simulink model "aeromissile_la"  (R2019b)
settings: Solver=ode45  StartTime=0.0  StopTime=20  RelTol=1e-3  EnableMultiTasking=on
PreLoadFcn:
  | aeromissile_la_dat
values from neighbouring files (symbols this model uses):
  cy_el = 0.034000/d2r    (= 1.94805650344)    [aeromissile_la_dat.m]
  cz_el = -0.034000/d2r    (= -1.94805650344)    [aeromissile_la_dat.m]
  d_ref = 0.2286    [aeromissile_la_dat.m]
  eul_0 = [0;0;0]    [aeromissile_la_dat.m]
  fin_max = 30.0*d2r    (= 0.523598775598)    [aeromissile_la_dat.m]
  fin_min = -30.0*d2r    (= -0.523598775598)    [aeromissile_la_dat.m]
  g = 9.81    [aeromissile_la_dat.m]
  inertia = inertia_0/2    [aeromissile_la_dat.m]
  inertia_0 = diag([Ixx Iyy Izz])    [aeromissile_la_dat.m]
  l_acc = 0.5    [aeromissile_la_dat.m]
  l_ref = 0.04    [aeromissile_la_dat.m]
  len_missile = 3    [aeromissile_la_dat.m]
  mass_0 = 234.02    [aeromissile_la_dat.m]
  massf = 30    [aeromissile_la_dat.m]
  mx_el = -0.206000/d2r    (= -11.8029305797)    [aeromissile_la_dat.m]
  mx_wx = -0.5    [aeromissile_la_dat.m]
  my_el = -0.206000/d2r    (= -11.8029305797)    [aeromissile_la_dat.m]
  my_wy = -1.719    [aeromissile_la_dat.m]
  mz_el = -0.206000/d2r    (= -11.8029305797)    [aeromissile_la_dat.m]
  mz_wz = -1.719    [aeromissile_la_dat.m]
  q = 2    [aeromissile_la_dat.m]
  S_ref = 0.040877    [aeromissile_la_dat.m]
  Thrust = 10e3    (= 10000)    [aeromissile_la_dat.m]
  Vm_0 = [300;0;0]    [aeromissile_la_dat.m]
  wm_0 = [0;0;0]    [aeromissile_la_dat.m]
  x_cg = 0.555*len_missile    (= 1.665)    [aeromissile_la_dat.m]
  x_cg_0 = 0.575*len_missile    (= 1.725)    [aeromissile_la_dat.m]
  x_ref = 0.54*len_missile    (= 1.62)    [aeromissile_la_dat.m]
  xmg_0 = [0;1000;0]    [aeromissile_la_dat.m]
undefined symbols (not defined in the file or in its folder): Earth, inv_fcn, WGS84
libraries: simulink_need_slupdate x26, sharedutil x3, aerolibobsolete x2, aerolibtransform2 x2, aerolibfltsims x2, aerolibprivatev1p5 x1, vrlib x1
(part 1 of 2)
settings Model: EnablePacing=on  Creator=Semen  LastModifiedBy=Semen
settings DataIOCC: LimitDataPoints=on  SaveFormat=Array  ReturnWorkspaceOutputs=off  SignalLoggingName=sigsOut
settings DebuggingCC: SaveWithParameterizedLinksMsg=none  UnderspecifiedInitializationDetection=Classic  MergeDetectMultiDrivingBlocksExec=none  SignalResolutionControl=TryResolveAllWithWarning  MultiTaskDSMMsg=warning  MultiTaskCondExecSysMsg=none
settings HardwareCC: ProdBitPerPointer=32  ProdBitPerSizeT=32  ProdBitPerPtrDiffT=32  ProdLargestAtomicFloat=None  ProdIntDivRoundTo=Undefined  ProdEndianess=Unspecified  ProdWordSize=32  ProdHWDeviceType=32-bit Generic  TargetUnknown=on
settings ModelReferenceCC: PropagateSignalLabelsOutOfModel=off
settings GRTTargetCC: CombineOutputUpdateFcns=off  GRTInterface=on
settings ConfigComp: CovMetricSettings=dw  CovHtmlReporting=on  CovSaveCumulativeToWorkspaceVar=on  CovSaveSingleToWorkspaceVar=on

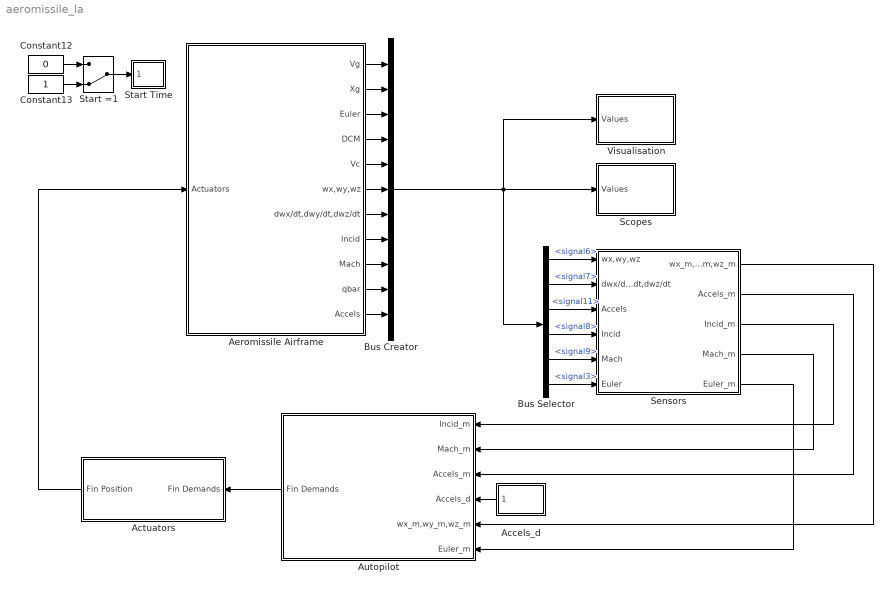
== system aeromissile_la ==
  Accels_d : Subsystem
  Actuators : Subsystem
  Aeromissile Airframe : Subsystem
  Autopilot : Subsystem
  Bus Creator : BusCreator  Inputs=11
  Bus Selector : BusSelector  OutputSignals=signal6,signal7,signal11,signal8,signal9,signal3
  Constant12 : Constant  Value=0  VectorParams1D=off
  Constant13 : Constant  VectorParams1D=off
  Scopes : Subsystem
  Sensors : Subsystem
  Start =1 : ManualSwitch  CurrentSetting=0
  Start Time : Subsystem
  Visualisation : Subsystem
  wires:
  Sensors/1(wx_m,wy_m,wz_m) -> Autopilot/5(wx_m,wy_m,wz_m)
  Sensors/2(Accels_m) -> Autopilot/3(Accels_m)
  Aeromissile Airframe/1(Vg) -> Bus Creator/1
  Aeromissile Airframe/2(Xg) -> Bus Creator/2
  Aeromissile Airframe/3(Euler) -> Bus Creator/3
  Aeromissile Airframe/4(DCM) -> Bus Creator/4
  Aeromissile Airframe/5(Vc) -> Bus Creator/5
  Aeromissile Airframe/6(wx,wy,wz) -> Bus Creator/6
  Aeromissile Airframe/7(dwx/dt,dwy/dt,dwz/dt) -> Bus Creator/7
  Aeromissile Airframe/11(Accels) -> Bus Creator/11
  Bus Selector/1 -> Sensors/1(wx,wy,wz)  "<signal6>"
  Bus Selector/2 -> Sensors/2(dwx/dt,dwy/dt,dwz/dt)  "<signal7>"
  Bus Selector/3 -> Sensors/3(Accels)  "<signal11>"
  Aeromissile Airframe/8(Incid) -> Bus Creator/8
  Aeromissile Airframe/10(qbar) -> Bus Creator/10
  Actuators/1(Fin Position) -> Aeromissile Airframe/1(Actuators)
  Sensors/3(Incid_m) -> Autopilot/1(Incid_m)
  Sensors/4(Mach_m) -> Autopilot/2(Mach_m)
  Bus Selector/4 -> Sensors/4(Incid)  "<signal8>"
  Bus Selector/5 -> Sensors/5(Mach)  "<signal9>"
  Bus Selector/6 -> Sensors/6(Euler)  "<signal3>"
  Sensors/5(Euler_m) -> Autopilot/6(Euler_m)
  Constant13/1 -> Start =1/2
  Constant12/1 -> Start =1/1
  Bus Creator/1 -> Visualisation/1(Values), Scopes/1(Values), Bus Selector/1
  Aeromissile Airframe/9(Mach) -> Bus Creator/9
  Start =1/1 -> Start Time/1(Start)
  Autopilot/1(Fin Demands) -> Actuators/1(Fin Demands)
  Accels_d/1("Accels_d ") -> Autopilot/4(Accels_d)

== system aeromissile_la/Accels_d ==
  Accels_d : Constant  Value=[0 g 1]  VectorParams1D=off
  Accels_dD : Constant  Value=[0 0 0]  VectorParams1D=off
  Switch : Switch  Criteria=u2 ~= 0  SaturateOnIntegerOverflow=on
  "Accels_d " : Outport
  wires:
  Switch/1 -> "Accels_d "/1
  Accels_dD/1 -> Switch/3
  [tD] -> Switch/2
  Accels_d/1 -> Switch/1

== system aeromissile_la/Actuators ==
  Fin Demands : Inport
  Lock Fin : Subsystem
  Second Order Nonlinear Actuator : aerolibobsolete/Second Order Nonlinear Actuator  wn_fin=wn_fin  z_fin=z_fin  fin_max=fin_max  fin_min=fin_min  fin_maxrate=fin_maxrate  fin_act_0=fin_act_0
      settings: SourceProductName=Aerospace Blockset  SourceProductBaseCode=AE
  Fin Position : Outport
  wires:
  Fin Demands/1 -> Lock Fin/1(FD)
  Second Order Nonlinear Actuator/1 -> Fin Position/1
  Lock Fin/1("FD ") -> Second Order Nonlinear Actuator/1

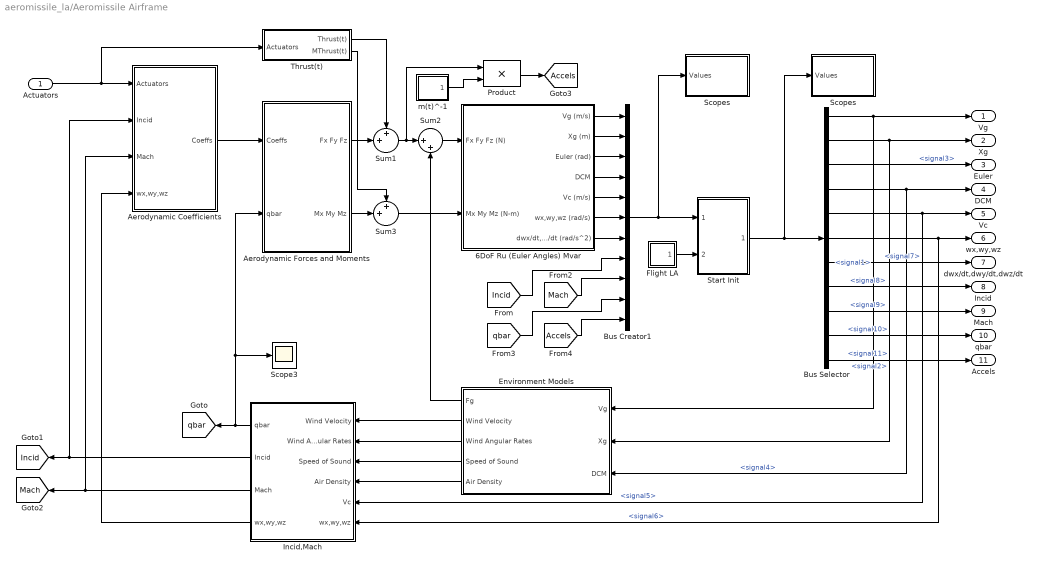
== system aeromissile_la/Aeromissile Airframe ==
  Actuators : Inport
  6DoF Ru (Euler Angles) Mvar : Subsystem  AncestorBlock=aerolib6dof/6DoF (Euler Angles)  mask(6DoF Ru (Euler Angles) EoM){xmg_0=xmg_0, Vm_0=Vm_0, eul_0=eul_0, wm_0=wm_0, mass_0=mass_0, massf=massf, q=q, inertia_0=inertia_0, inertia=inertia}
      mask prompts: xmg_0 "Initial position in inertial axes [Xg,Yg,Zg] (m):"; Vm_0 "Initial velocity in body axes [Vxc,Vyc,Vzc] (m/s):"; eul_0 "Initial Euler orientation [roll, pitch, yaw] (rad):"; wm_0 "Initial body rotation rates [wx,wy,wz] (rad/s):"; mass_0 "Initial mass(kg):"; massf "Mass of fuel (kg):"; q "Consumption of fuel (kg/s):"; inertia_0 "Initial inertia matrix (kg*m^2):"; inertia "Finite inertia matrix (kg*m^2)"
      mask help:
      | Integrate the six-degrees-of-freedom equations of motion using an Euler angle representation for the orientation of the body in space.
      |
      | Inputs are forces on the body in x-axis, y-axis, and z-axis; and moments on the body along x-axis, y-axis, and z-axis. Outputs are translational velocity in x-axis, y-axis, and z-axis in inertial coordinates; position in x-axis, y-axis, and z-axis in inertial coordinates; gamma, theta, and psi; 3-by-3 direction cosine matrix; translational velocity in x-axis, y-axis, and z-axis in body coordinates; roll, pitch, and yaw rate; and roll, pitch, and yaw acceleration.
      mask Display: disp('Euler\nAngles')
  Aerodynamic Coefficients : Subsystem
  Aerodynamic Forces and Moments : Subsystem  AncestorBlock=aeroblk_lib_HL20/HL20 Airframe/Forces and Moments
  Bus Creator1 : BusCreator  Inputs=11
  Bus Selector : BusSelector  OutputSignals=signal1,signal2,signal3,signal4,signal5,signal6,signal7,signal8,signal9,signal10,signal11
  Environment Models : Subsystem
  Flight LA : Subsystem
  Incid,Mach : Subsystem
  Product : Product  SaturateOnIntegerOverflow=on  OutDataTypeStr=Inherit: Same as first input
  Scope3 : Scope
  Scopes : Subsystem
  "Scopes " : Subsystem
  Start Init : Subsystem
  Sum1 : Sum  Inputs=++|  SaturateOnIntegerOverflow=on
  Sum2 : Sum  Inputs=|++  SaturateOnIntegerOverflow=on
  Sum3 : Sum  Inputs=++|  SaturateOnIntegerOverflow=on
  Thrust(t) : Subsystem
  m(t)^-1 : Subsystem
  Vg : Outport
  Xg : Outport  Port=2
  Euler : Outport  Port=3
  DCM : Outport  Port=4
  Vc : Outport  Port=5
  wx,wy,wz : Outport  Port=6
  dwx/dt,dwy/dt,dwz/dt : Outport  Port=7
  Incid : Outport  Port=8
  Mach : Outport  Port=9
  qbar : Outport  Port=10
  Accels : Outport  Port=11
  tag scope: Accels=global, Incid=global, Mach=global, qbar=global
  wires:
  Aerodynamic Coefficients/1(Coeffs) -> Aerodynamic Forces and Moments/1(Coeffs)
  Actuators/1 -> Aerodynamic Coefficients/1(Actuators), Thrust(t)/1(Actuators)
  Environment Models/1(Fg) -> Sum2/2
  Incid,Mach/1(qbar) -> Aerodynamic Forces and Moments/2(qbar), Scope3/1, [qbar]
  Incid,Mach/2(Incid) -> Aerodynamic Coefficients/2(Incid), [Incid]
  Incid,Mach/3(Mach) -> Aerodynamic Coefficients/3(Mach), [Mach]
  Incid,Mach/4("wx,wy,wz ") -> Aerodynamic Coefficients/4(wx,wy,wz)
  Environment Models/2(Wind Velocity) -> Incid,Mach/1(Wind Velocity)
  Environment Models/3(Wind Angular Rates) -> Incid,Mach/2(Wind Angular Rates)
  Environment Models/4(Speed of Sound) -> Incid,Mach/3(Speed of Sound)
  Environment Models/5(Air Density) -> Incid,Mach/4(Air Density)
  Aerodynamic Forces and Moments/1(Fx Fy Fz) -> Sum1/2
  Sum1/1 -> Sum2/1, Product/1
  m(t)^-1/1(m(t)^-1) -> Product/2
  6DoF Ru (Euler Angles) Mvar/1(Vg (m/s)) -> Bus Creator1/1
  6DoF Ru (Euler Angles) Mvar/2(Xg (m)) -> Bus Creator1/2
  6DoF Ru (Euler Angles) Mvar/3(Euler (rad)) -> Bus Creator1/3
  6DoF Ru (Euler Angles) Mvar/4(DCM) -> Bus Creator1/4
  6DoF Ru (Euler Angles) Mvar/5(Vc (m/s)) -> Bus Creator1/5
  6DoF Ru (Euler Angles) Mvar/6(wx,wy,wz (rad/s)) -> Bus Creator1/6
  6DoF Ru (Euler Angles) Mvar/7(dwx/dt,dwy/dt,dwz/dt (rad/s^2)) -> Bus Creator1/7
  Bus Selector/1 -> Vg/1, Environment Models/1(Vg)  "<signal1>"
  Bus Selector/2 -> Xg/1, Environment Models/2(Xg)  "<signal2>"
  Bus Selector/3 -> Euler/1  "<signal3>"
  Bus Selector/4 -> DCM/1, Environment Models/3(DCM)  "<signal4>"
  Bus Selector/5 -> Vc/1, Incid,Mach/5(Vc)  "<signal5>"
  Bus Selector/6 -> wx,wy,wz/1, Incid,Mach/6(wx,wy,wz)  "<signal6>"
  Bus Selector/7 -> dwx/dt,dwy/dt,dwz/dt/1  "<signal7>"
  Product/1 -> [Accels]
  Bus Selector/8 -> Incid/1  "<signal8>"
  Bus Selector/9 -> Mach/1  "<signal9>"
  Bus Selector/10 -> qbar/1  "<signal10>"
  Bus Selector/11 -> Accels/1  "<signal11>"
  [Incid] -> Bus Creator1/8
  [Mach] -> Bus Creator1/9
  [qbar] -> Bus Creator1/10
  [Accels] -> Bus Creator1/11
  Bus Creator1/1 -> Start Init/1("val_m "), Scopes/1(Values)
  Start Init/1(val_m) -> Bus Selector/1, "Scopes "/1(Values)
  Flight LA/1(val_la) -> Start Init/2("val_la ")
  Sum2/1 -> 6DoF Ru (Euler Angles) Mvar/1(Fx Fy Fz (N))
  Aerodynamic Forces and Moments/2(Mx My Mz) -> Sum3/2
  Sum3/1 -> 6DoF Ru (Euler Angles) Mvar/2(Mx My Mz (N-m))
  Thrust(t)/2(MThrust(t)) -> Sum3/1
  Thrust(t)/1(Thrust(t)) -> Sum1/1

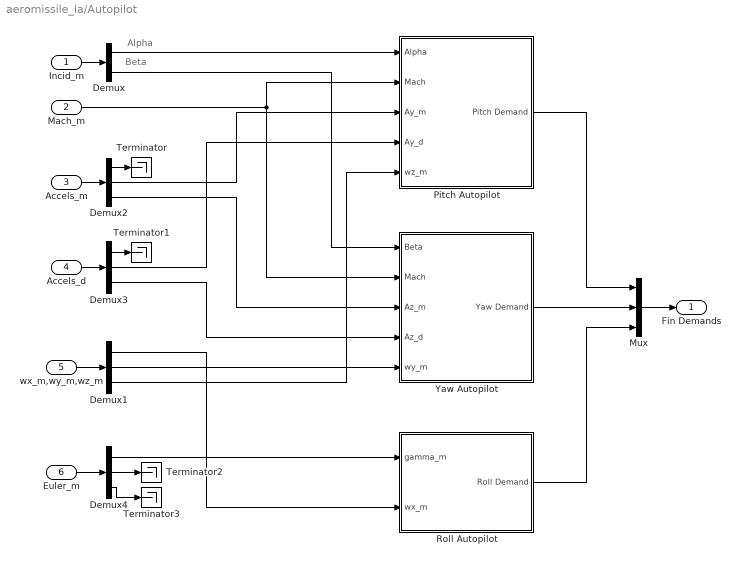
== system aeromissile_la/Autopilot ==
  note: Alpha
  note: Beta
  Incid_m : Inport
  Mach_m : Inport  Port=2
  Accels_m : Inport  Port=3
  Accels_d : Inport  Port=4
  wx_m,wy_m,wz_m : Inport  Port=5
  Euler_m : Inport  Port=6
  Demux : Demux  Outputs=2
  Demux{1..4} (4 alike) : Demux  Outputs=3
  Mux : Mux  Inputs=3
  Pitch Autopilot : Subsystem
  Roll Autopilot : Subsystem
  Terminator{,1..3} (4 alike) : Terminator
  Yaw Autopilot : Subsystem
  Fin Demands : Outport
  wires:
  Accels_m/1 -> Demux2/1
  Accels_d/1 -> Demux3/1
  Demux2/1 -> Terminator/1
  Demux3/1 -> Terminator1/1
  Incid_m/1 -> Demux/1
  Demux/1 -> Pitch Autopilot/1(Alpha)
  Demux/2 -> Yaw Autopilot/1(Beta)
  Demux2/2 -> Pitch Autopilot/3(Ay_m)
  Demux2/3 -> Yaw Autopilot/3(Az_m)
  Demux3/2 -> Pitch Autopilot/4(Ay_d)
  wx_m,wy_m,wz_m/1 -> Demux1/1
  Demux1/3 -> Pitch Autopilot/5(wz_m)
  Mach_m/1 -> Pitch Autopilot/2(Mach), Yaw Autopilot/2(Mach)
  Demux1/1 -> Roll Autopilot/2(wx_m)
  Demux3/3 -> Yaw Autopilot/4(Az_d)
  Demux1/2 -> Yaw Autopilot/5(wy_m)
  Pitch Autopilot/1(Pitch Demand) -> Mux/1
  Yaw Autopilot/1(Yaw Demand) -> Mux/2
  Roll Autopilot/1(Roll Demand) -> Mux/3
  Mux/1 -> Fin Demands/1
  Euler_m/1 -> Demux4/1
  Demux4/2 -> Terminator2/1
  Demux4/3 -> Terminator3/1
  Demux4/1 -> Roll Autopilot/1(gamma_m)

== system aeromissile_la/Scopes ==
  note: Vg
  note: Xg
  note: Euler
  note: DCM
  note: Vc
  note: wx,wy,wz
  note: dwx/dt,dwy/dt,
      | dwz/dt
  note: Incid
  note: Mach
  note: qbar
  note: Accels
  Values : Inport
  Bus Selector : BusSelector  OutputSignals=signal1,signal2,signal3,signal4,signal5,signal6,signal7,signal8,signal9,signal10,signal11
  Scope{1..11} (11 alike) : Scope
  wires:
  Bus Selector/1 -> Scope2/1  "<signal1>"
  Bus Selector/2 -> Scope1/1  "<signal2>"
  Bus Selector/3 -> Scope4/1  "<signal3>"
  Bus Selector/11 -> Scope11/1  "<signal11>"
  Bus Selector/10 -> Scope10/1  "<signal10>"
  Bus Selector/9 -> Scope9/1  "<signal9>"
  Bus Selector/8 -> Scope8/1  "<signal8>"
  Bus Selector/7 -> Scope7/1  "<signal7>"
  Bus Selector/6 -> Scope6/1  "<signal6>"
  Bus Selector/5 -> Scope5/1  "<signal5>"
  Bus Selector/4 -> Scope3/1  "<signal4>"
  Values/1 -> Bus Selector/1

== system aeromissile_la/Sensors ==
  note: Rate Gyro
  wx,wy,wz : Inport
  dwx/dt,dwy/dt,dwz/dt : Inport  Port=2
  Accels : Inport  Port=3
  Incid : Inport  Port=4
  Mach : Inport  Port=5
  Euler : Inport  Port=6
  Demux : Demux  Outputs=3
  Demux1 : Demux  Outputs=3
  Gain : Gain  Gain=l_acc  SaturateOnIntegerOverflow=on  OutDataTypeStr=Inherit: Same as input  ParamDataTypeStr=Inherit: Same as input
  Mux : Mux  Inputs=3
  Sum : Sum  Inputs=-+|  SaturateOnIntegerOverflow=on
  Sum1 : Sum  Inputs=++|  SaturateOnIntegerOverflow=on
  Tminator1 : Terminator
  wx_m,wy_m,wz_m : Outport
  Accels_m : Outport  Port=2
  Incid_m : Outport  Port=3
  Mach_m : Outport  Port=4
  Euler_m : Outport  Port=5
  wires:
  wx,wy,wz/1 -> wx_m,wy_m,wz_m/1
  dwx/dt,dwy/dt,dwz/dt/1 -> Gain/1
  Accels/1 -> Demux/1
  Demux/1 -> Mux/1
  Gain/1 -> Demux1/1
  Demux/3 -> Sum/2
  Demux1/2 -> Sum/1
  Demux1/1 -> Tminator1/1
  Sum/1 -> Mux/3
  Mux/1 -> Accels_m/1  "Accelerometer"
  Demux/2 -> Sum1/2
  Demux1/3 -> Sum1/1
  Sum1/1 -> Mux/2
  Incid/1 -> Incid_m/1
  Mach/1 -> Mach_m/1
  Euler/1 -> Euler_m/1

== system aeromissile_la/Start Time ==
  Start : Inport
  t departure : Subsystem
  t engine : Subsystem
  t start : Subsystem
  tag scope: Start=global, tD=global, tE=global, tS=global
  wires:
  t start/1(tS) -> t engine/1(tS), [tS], t departure/1(tS)
  t engine/1(tE) -> [tE]
  t departure/1(tD) -> [tD]
  Start/1 -> t start/1(S), [Start]

== system aeromissile_la/Visualisation ==
  note: Euler
  note: Xg
  Values : Inport
  Bus Selector : BusSelector  OutputSignals=signal2,signal3
  FlightGear Animation : Subsystem
  Scope1 : Scope
  Scope4 : Scope
  VR Sink Animation : Subsystem
  wires:
  Bus Selector/2 -> FlightGear Animation/2(Euler), Scope4/1, VR Sink Animation/2(Euler)  "<signal3>"
  Bus Selector/1 -> VR Sink Animation/1(Xg), FlightGear Animation/1(Xg), Scope1/1  "<signal2>"
  Values/1 -> Bus Selector/1

== system aeromissile_la/Actuators/Lock Fin ==
  FD : Inport
  Constant6 : Constant  Value=[0; 0; 0]  VectorParams1D=off
  Switch : Switch  Criteria=u2 ~= 0  SaturateOnIntegerOverflow=on
  "FD " : Outport
  wires:
  FD/1 -> Switch/1
  Switch/1 -> "FD "/1
  [Start] -> Switch/2
  Constant6/1 -> Switch/3

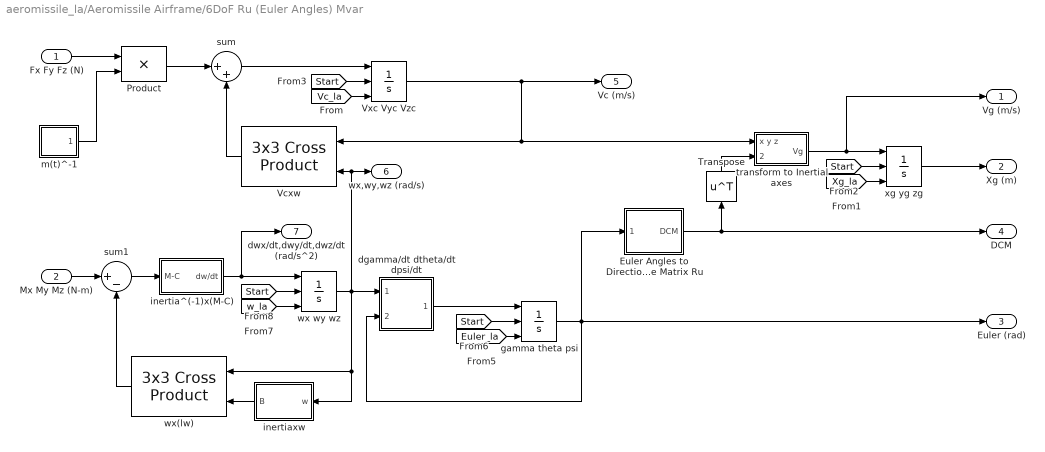
== system aeromissile_la/Aeromissile Airframe/6DoF Ru (Euler Angles) Mvar ==
  Fx Fy Fz (N) : Inport
  Mx My Mz (N-m) : Inport  Port=2
  Euler Angles to Direction Cosine Matrix Ru : Subsystem  AncestorBlock="aerolibtransform/Euler Angles to  Direction Cosine Matrix"  mask(Euler2DCM){}
      mask help: Determine the 3-by-3 direction cosine matrix (DCM) from an Euler orientation (roll, pitch, yaw). The output DCM transforms vectors from inertial axes to body axes.
      mask Help: web(asbhelp('euleranglestodirectioncosinematrix'));
      mask Display: disp('Eul2DCM')
  Product : Product  SaturateOnIntegerOverflow=on  OutDataTypeStr=Inherit: Same as first input
  Transpose : Math  Operator=transpose  SaturateOnIntegerOverflow=on
  Vcxw : sharedutil/3x3 Cross Product  aMode=aMode
      settings: SourceProductBaseCode=AE
  Vxc Vyc Vzc : Integrator  ExternalReset=either  InitialConditionSource=external  InitialCondition=Vm_0
  dgamma/dt dtheta/dt dpsi/dt : Subsystem
  gamma theta psi : Integrator  ExternalReset=either  InitialConditionSource=external  InitialCondition=Vm_0
  inertia^(-1)x(M-C) : Subsystem
  inertiaxw : Subsystem
  m(t)^-1 : Subsystem
  sum : Sum  Inputs=|++  SaturateOnIntegerOverflow=on  InputSameDT=on  OutDataTypeStr=Inherit: Same as first input
  sum1 : Sum  Inputs=|+-  SaturateOnIntegerOverflow=on  InputSameDT=on  OutDataTypeStr=Inherit: Same as first input
  "transform to Inertial axes " : Subsystem  mask(Vector Transformation){}
      mask Display: disp('L_EB')
  wx wy wz : Integrator  ExternalReset=either  InitialConditionSource=external  InitialCondition=Vm_0
  wx(lw) : sharedutil/3x3 Cross Product  aMode=aMode
      settings: SourceProductBaseCode=AE
  xg yg zg : Integrator  ExternalReset=either  InitialConditionSource=external  InitialCondition=Vm_0
  Vg (m/s) : Outport
  Xg (m) : Outport  Port=2
  Euler (rad) : Outport  Port=3
  DCM : Outport  Port=4
  Vc (m/s) : Outport  Port=5
  wx,wy,wz (rad/s) : Outport  Port=6
  dwx/dt,dwy/dt,dwz/dt (rad/s^2) : Outport  Port=7
  wires:
  Transpose/1 -> "transform to Inertial axes "/2(transform coefficients)
  Euler Angles to Direction Cosine Matrix Ru/1(DCM) -> Transpose/1, DCM/1
  Product/1 -> sum/1
  Vcxw/1 -> sum/2
  Fx Fy Fz (N)/1 -> Product/1
  inertia^(-1)x(M-C)/1(dw/dt) -> dwx/dt,dwy/dt,dwz/dt (rad/s^2)/1, wx wy wz/1
  wx(lw)/1 -> sum1/2
  inertiaxw/1(B) -> wx(lw)/2
  Mx My Mz (N-m)/1 -> sum1/1
  sum1/1 -> inertia^(-1)x(M-C)/1(M-C)
  wx wy wz/1 -> Vcxw/2, wx,wy,wz (rad/s)/1, wx(lw)/1, inertiaxw/1(w), dgamma/dt dtheta/dt dpsi/dt/1(wx wy wz)
  "transform to Inertial axes "/1(Vg) -> Vg (m/s)/1, xg yg zg/1
  xg yg zg/1 -> Xg (m)/1
  Vxc Vyc Vzc/1 -> "transform to Inertial axes "/1(x y z), Vcxw/1, Vc (m/s)/1
  gamma theta psi/1 -> dgamma/dt dtheta/dt dpsi/dt/2(gamma theta psi), Euler Angles to Direction Cosine Matrix Ru/1(Euler Roll Pitch Yaw), Euler (rad)/1
  dgamma/dt dtheta/dt dpsi/dt/1(dgamma/dt dtheta/dt dpsi/dt) -> gamma theta psi/1
  m(t)^-1/1(m(t)^-1) -> Product/2
  [Start] -> xg yg zg/2
  [Xg_la] -> xg yg zg/3
  sum/1 -> Vxc Vyc Vzc/1
  [Start] -> Vxc Vyc Vzc/2
  [Vc_la] -> Vxc Vyc Vzc/3
  [Euler_la] -> gamma theta psi/3
  [Start] -> wx wy wz/2
  [w_la] -> wx wy wz/3
  [Start] -> gamma theta psi/2

== system aeromissile_la/Aeromissile Airframe/Aerodynamic Coefficients ==
  Actuators : Inport
  Incid : Inport  Port=2
  Mach : Inport  Port=3
  wx,wy,wz : Inport  Port=4
  Actuator Increments : Subsystem
  Body Rate Damping : Subsystem
  Cross Link Coefficients : Subsystem
  Datum Coefficients : Subsystem
  Sum : Sum  Inputs=++++  SaturateOnIntegerOverflow=on
  Coeffs : Outport  InitialOutput=[0]
  wires:
  Mach/1 -> Datum Coefficients/2(Mach), Cross Link Coefficients/2(Mach)
  Actuators/1 -> Actuator Increments/1(Actuator Deflections), Cross Link Coefficients/3(Actuators)
  Incid/1 -> Datum Coefficients/1(Incid), Cross Link Coefficients/1(Incid)
  Datum Coefficients/1(Datum Coeffs) -> Sum/1
  Actuator Increments/1(Actuator Coeffs) -> Sum/2
  Sum/1 -> Coeffs/1
  wx,wy,wz/1 -> Body Rate Damping/1(wx,wy,wz)
  Body Rate Damping/1(Damping Coeffs) -> Sum/4
  Cross Link Coefficients/1(Cross Coeffs) -> Sum/3

== system aeromissile_la/Aeromissile Airframe/Aerodynamic Forces and Moments ==
  Coeffs : Inport
  qbar : Inport  Port=2
  3x3 Cross Product : sharedutil/3x3 Cross Product  aMode=aMode
      settings: SourceProductBaseCode=AE
  Demux1 : Demux  Outputs=[3,3]
  Gain : Gain  Gain=[-1 1 1]  SaturateOnIntegerOverflow=on  OutDataTypeStr=Inherit: Same as input  ParamDataTypeStr=Inherit: Same as input
  Moments about Centre of Gravity : Subsystem
  Product : Product  SaturateOnIntegerOverflow=on  InputSameDT=on  OutDataTypeStr=Inherit: Same as first input
  Product3 : Product  SaturateOnIntegerOverflow=on  InputSameDT=on  OutDataTypeStr=Inherit: Same as first input
  Scope : Scope
  Sum1 : Sum  Inputs=++|  SaturateOnIntegerOverflow=on  InputSameDT=on  OutDataTypeStr=Inherit: Same as first input
  reference area : Gain  Gain=S_ref  SaturateOnIntegerOverflow=on  OutDataTypeStr=Inherit: Same as input  ParamDataTypeStr=Inherit: Same as input
  reference length : Gain  Gain=[l_ref d_ref d_ref]  SaturateOnIntegerOverflow=on  OutDataTypeStr=Inherit: Same as input  ParamDataTypeStr=Inherit: Same as input
  Fx Fy Fz : Outport  InitialOutput=[0]
  Mx My Mz : Outport  Port=2  InitialOutput=[0]
  wires:
  Sum1/1 -> Mx My Mz/1
  Product3/1 -> Sum1/2
  Moments about Centre of Gravity/1(-(x_cg-x_ref)) -> 3x3 Cross Product/2, Scope/1
  Product/1 -> 3x3 Cross Product/1, Fx Fy Fz/1
  reference area/1 -> reference length/1, Gain/1
  qbar/1 -> reference area/1
  Demux1/2 -> Product3/1  "mx my mz"
  Demux1/1 -> Product/1  "cx cy cz"
  Coeffs/1 -> Demux1/1
  reference length/1 -> Product3/2
  3x3 Cross Product/1 -> Sum1/1
  Gain/1 -> Product/2

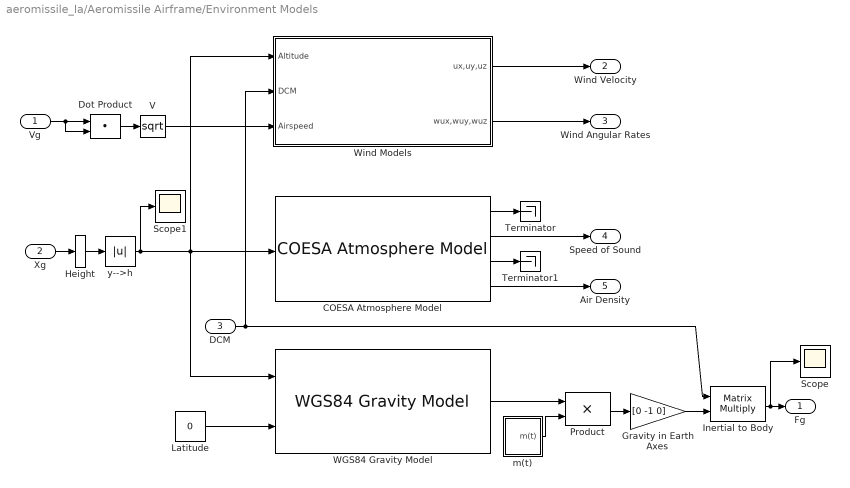
== system aeromissile_la/Aeromissile Airframe/Environment Models ==
  Vg : Inport
  Xg : Inport  Port=2
  DCM : Inport  Port=3
  COESA Atmosphere Model : aerolibprivatev1p5/COESA Atmosphere Model  units=Metric
      settings: SourceProductName=Aerospace Blockset  SourceProductBaseCode=AE
  Dot Product : DotProduct  InputSameDT=on  OutDataTypeStr=Inherit: Inherit via internal rule
  Gravity in Earth Axes : Gain  Gain=[0 -1 0]  SaturateOnIntegerOverflow=on  OutDataTypeStr=Inherit: Same as input  ParamDataTypeStr=Inherit: Same as input
  Height : Selector  InputPortWidth=3  IndexOptions=Index vector (dialog)  Indices=[2]  OutputSizes=1
  Inertial to Body : Product  Multiplication=Matrix(*)  SaturateOnIntegerOverflow=on  InputSameDT=on  OutDataTypeStr=Inherit: Same as first input
  Latitude : Constant  Value=0
  Product : Product  SaturateOnIntegerOverflow=on  OutDataTypeStr=Inherit: Same as first input
  Scope : Scope
  Scope1 : Scope
  Terminator : Terminator
  Terminator1 : Terminator
  V : Math  Operator=sqrt  SaturateOnIntegerOverflow=on
  WGS84 Gravity Model : aerolibobsolete/WGS84 Gravity Model  model=WGS84 Taylor Series  units=Metric (MKS)  no_atmos=on  precessing=on  month=February  day=1  year=2000  no_centrifugal=on  action=Warning
      settings: SourceProductName=Aerospace Blockset  SourceProductBaseCode=AE
  Wind Models : Subsystem
  m(t) : Subsystem
  y-->h : Abs  SaturateOnIntegerOverflow=on
  Fg : Outport
  Wind Velocity : Outport  Port=2
  Wind Angular Rates : Outport  Port=3
  Speed of Sound : Outport  Port=4
  Air Density : Outport  Port=5
  wires:
  Latitude/1 -> WGS84 Gravity Model/2
  COESA Atmosphere Model/1 -> Terminator/1
  COESA Atmosphere Model/3 -> Terminator1/1
  Wind Models/1(ux,uy,uz) -> Wind Velocity/1
  Wind Models/2(wux,wuy,wuz) -> Wind Angular Rates/1
  COESA Atmosphere Model/2 -> Speed of Sound/1
  COESA Atmosphere Model/4 -> Air Density/1
  Height/1 -> y-->h/1
  Xg/1 -> Height/1
  Vg/1 -> Dot Product/2, Dot Product/1
  Dot Product/1 -> V/1
  Gravity in Earth Axes/1 -> Inertial to Body/2
  Inertial to Body/1 -> Fg/1, Scope/1
  DCM/1 -> Wind Models/2(DCM), Inertial to Body/1
  y-->h/1 -> COESA Atmosphere Model/1, WGS84 Gravity Model/1, Wind Models/1(Altitude), Scope1/1
  V/1 -> Wind Models/3(Airspeed)
  WGS84 Gravity Model/1 -> Product/1
  Product/1 -> Gravity in Earth Axes/1
  m(t)/1(m(t)) -> Product/2

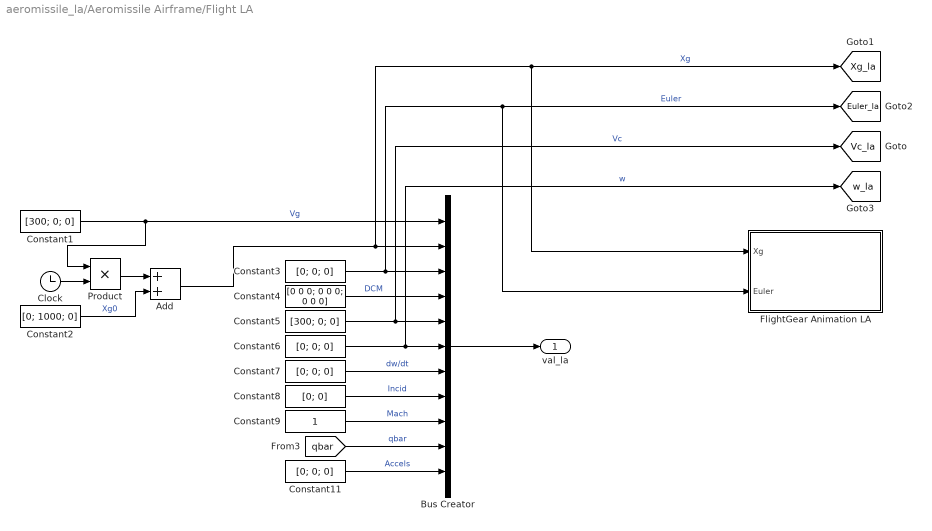
== system aeromissile_la/Aeromissile Airframe/Flight LA ==
  Add : Sum
  Bus Creator : BusCreator  Inputs=11
  Clock : Clock
  Constant1 : Constant  Value=[300; 0; 0]  VectorParams1D=off
  Constant{3,6..7,11} (4 alike) : Constant  Value=[0; 0; 0]  VectorParams1D=off
  Constant2 : Constant  Value=[0; 1000; 0]  VectorParams1D=off
  Constant4 : Constant  Value=[0 0 0; 0 0 0; 0 0 0]  VectorParams1D=off
  Constant5 : Constant  Value=[300; 0; 0]  VectorParams1D=off
  Constant8 : Constant  Value=[0; 0]  VectorParams1D=off
  Constant9 : Constant  VectorParams1D=off
  FlightGear Animation LA : Subsystem
  Product : Product
  val_la : Outport
  tag scope: Euler_la=global, Vc_la=global, Xg_la=global, w_la=global
  wires:
  Constant1/1 -> Product/1, Bus Creator/1  "Vg"
  Constant3/1 -> Bus Creator/3, FlightGear Animation LA/2(Euler), [Euler_la]  "Euler"
  Constant6/1 -> Bus Creator/6, [w_la]  "w"
  Constant7/1 -> Bus Creator/7  "dw/dt"
  Constant8/1 -> Bus Creator/8  "Incid"
  Constant9/1 -> Bus Creator/9  "Mach"
  [qbar] -> Bus Creator/10  "qbar"
  Constant11/1 -> Bus Creator/11  "Accels"
  Bus Creator/1 -> val_la/1
  Constant4/1 -> Bus Creator/4  "DCM"
  Constant5/1 -> Bus Creator/5, [Vc_la]  "Vc"
  Clock/1 -> Product/2
  Constant2/1 -> Add/2  "Xg0"
  Product/1 -> Add/1
  Add/1 -> FlightGear Animation LA/1(Xg), [Xg_la], Bus Creator/2  "Xg"

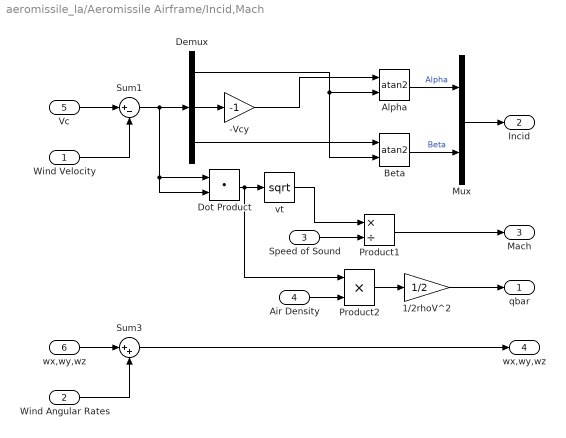
== system aeromissile_la/Aeromissile Airframe/Incid,Mach ==
  Wind Velocity : Inport
  Wind Angular Rates : Inport  Port=2
  Speed of Sound : Inport  Port=3
  Air Density : Inport  Port=4
  Vc : Inport  Port=5
  wx,wy,wz : Inport  Port=6
  -Vcy : Gain  Gain=-1  SaturateOnIntegerOverflow=on  OutDataTypeStr=Inherit: Same as input  ParamDataTypeStr=Inherit: Same as input
  1/2rhoV^2 : Gain  Gain=1/2  SaturateOnIntegerOverflow=on  OutDataTypeStr=Inherit: Same as input  ParamDataTypeStr=Inherit: Same as input
  Alpha : Trigonometry  Operator=atan2
  Beta : Trigonometry  Operator=atan2
  Demux : Demux  Outputs=3
  Dot Product : DotProduct  InputSameDT=on  OutDataTypeStr=Inherit: Inherit via internal rule
  Mux : Mux  Inputs=2
  Product1 : Product  Inputs=*/  SaturateOnIntegerOverflow=on  InputSameDT=on  OutDataTypeStr=Inherit: Same as first input
  Product2 : Product  SaturateOnIntegerOverflow=on  InputSameDT=on  OutDataTypeStr=Inherit: Same as first input
  Sum1 : Sum  Inputs=|+-  SaturateOnIntegerOverflow=on
  Sum3 : Sum  Inputs=|++  SaturateOnIntegerOverflow=on
  vt : Math  Operator=sqrt  SaturateOnIntegerOverflow=on
  qbar : Outport  InitialOutput=0
  Incid : Outport  Port=2
  Mach : Outport  Port=3
  "wx,wy,wz " : Outport  Port=4
  wires:
  1/2rhoV^2/1 -> qbar/1
  Product2/1 -> 1/2rhoV^2/1
  Air Density/1 -> Product2/2
  Dot Product/1 -> Product2/1, vt/1
  Product1/1 -> Mach/1
  vt/1 -> Product1/1
  Sum1/1 -> Dot Product/2, Dot Product/1, Demux/1
  Vc/1 -> Sum1/1
  Speed of Sound/1 -> Product1/2
  Wind Velocity/1 -> Sum1/2
  Demux/1 -> Alpha/2, Beta/2
  Beta/1 -> Mux/2  "Beta"
  Mux/1 -> Incid/1
  Alpha/1 -> Mux/1  "Alpha"
  wx,wy,wz/1 -> Sum3/1
  Wind Angular Rates/1 -> Sum3/2
  Sum3/1 -> "wx,wy,wz "/1
  Demux/2 -> -Vcy/1
  -Vcy/1 -> Alpha/1
  Demux/3 -> Beta/1

== system aeromissile_la/Aeromissile Airframe/Scopes ==
  note: Vg
  note: Xg
  note: Euler
  note: DCM
  note: Vc
  note: wx,wy,wz
  note: dwx/dt,dwy/dt,
      | dwz/dt
  note: Incid
  note: Mach
  note: qbar
  note: Accels
  Values : Inport
  Bus Selector : BusSelector  OutputSignals=signal1,signal2,signal3,signal4,signal5,signal6,signal7,signal8,signal9,signal10,signal11
  Scope{1..11} (11 alike) : Scope
  wires:
  Bus Selector/1 -> Scope2/1  "<signal1>"
  Bus Selector/2 -> Scope1/1  "<signal2>"
  Bus Selector/3 -> Scope4/1  "<signal3>"
  Bus Selector/11 -> Scope11/1  "<signal11>"
  Bus Selector/10 -> Scope10/1  "<signal10>"
  Bus Selector/9 -> Scope9/1  "<signal9>"
  Bus Selector/8 -> Scope8/1  "<signal8>"
  Bus Selector/7 -> Scope7/1  "<signal7>"
  Bus Selector/6 -> Scope6/1  "<signal6>"
  Bus Selector/5 -> Scope5/1  "<signal5>"
  Bus Selector/4 -> Scope3/1  "<signal4>"
  Values/1 -> Bus Selector/1

== system aeromissile_la/Aeromissile Airframe/Scopes  ==
  note: Vg
  note: Xg
  note: Euler
  note: DCM
  note: Vc
  note: wx,wy,wz
  note: dwx/dt,dwy/dt,
      | dwz/dt
  note: Incid
  note: Mach
  note: qbar
  note: Accels
  Values : Inport
  Bus Selector : BusSelector  OutputSignals=signal1,signal2,signal3,signal4,signal5,signal6,signal7,signal8,signal9,signal10,signal11
  Scope{1..11} (11 alike) : Scope
  wires:
  Bus Selector/1 -> Scope2/1  "<signal1>"
  Bus Selector/2 -> Scope1/1  "<signal2>"
  Bus Selector/3 -> Scope4/1  "<signal3>"
  Bus Selector/11 -> Scope11/1  "<signal11>"
  Bus Selector/10 -> Scope10/1  "<signal10>"
  Bus Selector/9 -> Scope9/1  "<signal9>"
  Bus Selector/8 -> Scope8/1  "<signal8>"
  Bus Selector/7 -> Scope7/1  "<signal7>"
  Bus Selector/6 -> Scope6/1  "<signal6>"
  Bus Selector/5 -> Scope5/1  "<signal5>"
  Bus Selector/4 -> Scope3/1  "<signal4>"
  Values/1 -> Bus Selector/1

== system aeromissile_la/Aeromissile Airframe/Start Init ==
  "val_m " : Inport
  "val_la " : Inport  Port=2
  Bus Creator : BusCreator  Inputs=11
  Bus Selector : BusSelector  OutputSignals=signal1,signal2,signal3,signal4,signal5,signal6,signal7,signal8,signal9,signal10,signal11
  Bus Selector1 : BusSelector  OutputSignals=Vg,Xg,Euler,DCM,Vc,w,dw/dt,Incid,Mach,qbar,Accels
  Demux : Demux  Outputs=2
  Mux1 : Mux  Inputs=2
  Mux2 : Mux  Inputs=2
  Subsystem : Subsystem
  Subsystem1 : Subsystem
  Subsystem2 : Subsystem
  Subsystem3 : Subsystem
  Subsystem4 : Subsystem
  Subsystem5 : Subsystem
  Subsystem6 : Subsystem
  Subsystem7 : Subsystem
  Subsystem8 : Subsystem
  Subsystem9 : Subsystem
  val_m : Outport
  wires:
  "val_m "/1 -> Bus Selector/1
  "val_la "/1 -> Bus Selector1/1
  Bus Selector/2 -> Subsystem1/1(Xg_m)  "<signal2>"
  Bus Selector/3 -> Subsystem7/1(Euler_m)  "<signal3>"
  Bus Selector/4 -> Subsystem2/1(DCM_m)  "<signal4>"
  Bus Selector/5 -> Subsystem8/1(Vc_m)  "<signal5>"
  Bus Selector/6 -> Subsystem3/1(w_m)  "<signal6>"
  Bus Selector/7 -> Subsystem4/1(dw/dt_m)  "<signal7>"
  Bus Selector1/10 -> Mux1/2  "<qbar>"
  Bus Selector1/9 -> Mux1/1  "<Mach>"
  Mux1/1 -> Subsystem9/2(M_q_la)
  Bus Selector1/8 -> Subsystem6/2(Incid_la)  "<Incid>"
  Bus Selector1/7 -> Subsystem4/2(dw/dt_la)  "<dw/dt>"
  Bus Selector1/6 -> Subsystem3/2(w_la)  "<w>"
  Bus Selector1/5 -> Subsystem8/2(Vc_la)  "<Vc>"
  Bus Selector1/4 -> Subsystem2/2(DCM_la)  "<DCM>"
  Bus Selector1/3 -> Subsystem7/2(Euler_la)  "<Euler>"
  Bus Selector1/2 -> Subsystem1/2(Xg_la)  "<Xg>"
  Subsystem9/1("M_q ") -> Demux/1
  Bus Creator/1 -> val_m/1
  Subsystem/1(Vg) -> Bus Creator/1
  Subsystem2/1("DCM ") -> Bus Creator/4
  Demux/1 -> Bus Creator/9
  Demux/2 -> Bus Creator/10
  Bus Selector/10 -> Mux2/2  "<signal10>"
  Bus Selector/9 -> Mux2/1  "<signal9>"
  Bus Selector/8 -> Subsystem6/1(Incid_m)  "<signal8>"
  Mux2/1 -> Subsystem9/1(M_q_m)
  Bus Selector/11 -> Subsystem5/1(Accels_m)  "<signal11>"
  Bus Selector1/1 -> Subsystem/2(Vg_la)  "<Vg>"
  Bus Selector/1 -> Subsystem/1(Vg_m)  "<signal1>"
  Subsystem1/1("Xg ") -> Bus Creator/2
  Subsystem7/1("Euler ") -> Bus Creator/3
  Subsystem8/1("Vc ") -> Bus Creator/5
  Subsystem3/1("w ") -> Bus Creator/6
  Subsystem4/1("dw/dt ") -> Bus Creator/7
  Subsystem6/1("Incid ") -> Bus Creator/8
  Bus Selector1/11 -> Subsystem5/2(Accels_la)  "<Accels>"
  Subsystem5/1("Accels ") -> Bus Creator/11

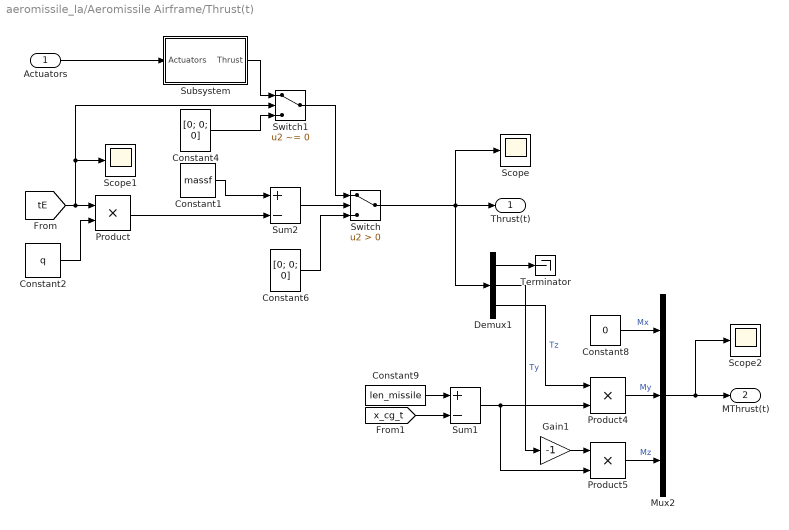
== system aeromissile_la/Aeromissile Airframe/Thrust(t) ==
  Actuators : Inport
  Constant1 : Constant  Value=massf
  Constant2 : Constant  Value=q
  Constant4 : Constant  Value=[0; 0; 0]  VectorParams1D=off
  Constant6 : Constant  Value=[0; 0; 0]  VectorParams1D=off
  Constant8 : Constant  Value=0
  Constant9 : Constant  Value=len_missile
  Demux1 : Demux  Outputs=3
  Gain1 : Gain  Gain=-1  SaturateOnIntegerOverflow=on  OutDataTypeStr=Inherit: Same as input  ParamDataTypeStr=Inherit: Same as input
  Mux2 : Mux  Inputs=3
  Product : Product  SaturateOnIntegerOverflow=on  OutDataTypeStr=Inherit: Same as first input
  Product4 : Product  SaturateOnIntegerOverflow=on  OutDataTypeStr=Inherit: Same as first input
  Product5 : Product  SaturateOnIntegerOverflow=on  OutDataTypeStr=Inherit: Same as first input
  Scope : Scope
  Scope1 : Scope
  Scope2 : Scope
  Subsystem : Subsystem
  Sum1 : Sum  Inputs=+-  SaturateOnIntegerOverflow=on
  Sum2 : Sum  Inputs=+-  SaturateOnIntegerOverflow=on
  Switch : Switch  Criteria=u2 > Threshold  SaturateOnIntegerOverflow=on
  Switch1 : Switch  Criteria=u2 ~= 0  SaturateOnIntegerOverflow=on
  Terminator : Terminator
  Thrust(t) : Outport
  MThrust(t) : Outport  Port=2
  wires:
  [tE] -> Product/1, Switch1/2, Scope1/1
  Constant2/1 -> Product/2
  Constant1/1 -> Sum2/1
  Product/1 -> Sum2/2
  Sum2/1 -> Switch/2
  Constant6/1 -> Switch/3
  Subsystem/1(Thrust) -> Switch1/1
  Constant4/1 -> Switch1/3
  Switch1/1 -> Switch/1
  Constant8/1 -> Mux2/1  "Mx"
  Product4/1 -> Mux2/2  "My"
  Constant9/1 -> Sum1/1
  [x_cg_t] -> Sum1/2
  Sum1/1 -> Product4/2, Product5/2
  Product5/1 -> Mux2/3  "Mz"
  Gain1/1 -> Product5/1
  Mux2/1 -> MThrust(t)/1, Scope2/1
  Actuators/1 -> Subsystem/1(Actuators)
  Switch/1 -> Demux1/1, Thrust(t)/1, Scope/1
  Demux1/1 -> Terminator/1
  Demux1/3 -> Product4/1  "Tz"
  Demux1/2 -> Gain1/1  "Ty"

== system aeromissile_la/Aeromissile Airframe/m(t)^-1 ==
  Constant : Constant  Value=mass_0
  Constant1 : Constant  Value=massf
  Constant2 : Constant  Value=q
  Constant3 : Constant  Value=-1
  Math Function : Math  Operator=pow  SaturateOnIntegerOverflow=on
  Product : Product  SaturateOnIntegerOverflow=on  OutDataTypeStr=Inherit: Same as first input
  Scope : Scope
  Sum2 : Sum  Inputs=|+-  SaturateOnIntegerOverflow=on
  Sum4 : Sum  Inputs=|+-  SaturateOnIntegerOverflow=on
  Sum5 : Sum  Inputs=|+-  SaturateOnIntegerOverflow=on
  Switch1 : Switch  Criteria=u2 > Threshold  SaturateOnIntegerOverflow=on
  m(t)^-1 : Outport
  wires:
  Constant2/1 -> Product/1
  [tE] -> Product/2
  Constant1/1 -> Sum2/1, Sum4/2
  Product/1 -> Sum2/2, Sum5/2
  Sum2/1 -> Switch1/2
  Sum4/1 -> Switch1/3
  Constant/1 -> Sum5/1, Sum4/1
  Sum5/1 -> Switch1/1
  Switch1/1 -> Scope/1, Math Function/1  "m(t)"
  Constant3/1 -> Math Function/2
  Math Function/1 -> m(t)^-1/1

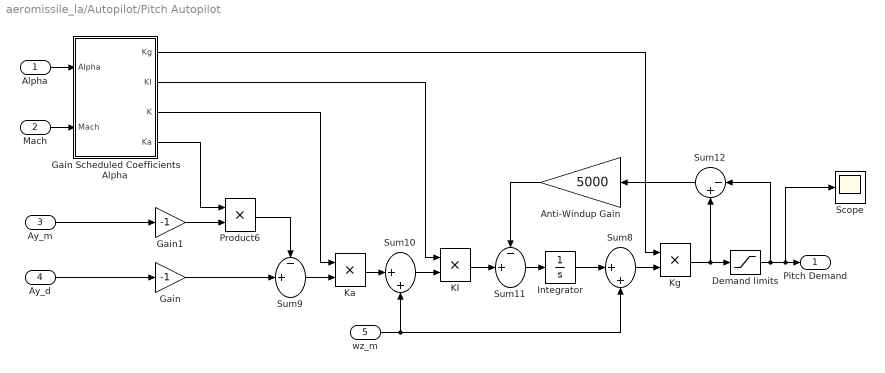
== system aeromissile_la/Autopilot/Pitch Autopilot ==
  Alpha : Inport
  Mach : Inport  Port=2
  Ay_m : Inport  Port=3
  Ay_d : Inport  Port=4
  wz_m : Inport  Port=5
  Anti-Windup Gain : Gain  Gain=5000  SaturateOnIntegerOverflow=on  OutDataTypeStr=Inherit: Same as input  ParamDataTypeStr=Inherit: Same as input
  "Demand limits " : Saturate  UpperLimit=fin_max  LowerLimit=fin_min
  Gain : Gain  Gain=-1  SaturateOnIntegerOverflow=on  OutDataTypeStr=Inherit: Same as input  ParamDataTypeStr=Inherit: Same as input
  Gain Scheduled Coefficients Alpha : Subsystem
  Gain1 : Gain  Gain=-1  SaturateOnIntegerOverflow=on  OutDataTypeStr=Inherit: Same as input  ParamDataTypeStr=Inherit: Same as input
  Integrator : Integrator
  KI : Product  SaturateOnIntegerOverflow=on  InputSameDT=on  OutDataTypeStr=Inherit: Same as first input
  Ka : Product  SaturateOnIntegerOverflow=on  InputSameDT=on  OutDataTypeStr=Inherit: Same as first input
  Kg : Product  SaturateOnIntegerOverflow=on  InputSameDT=on  OutDataTypeStr=Inherit: Same as first input
  Product6 : Product  SaturateOnIntegerOverflow=on  InputSameDT=on  OutDataTypeStr=Inherit: Same as first input
  Scope : Scope
  Sum10 : Sum  Inputs=|++  SaturateOnIntegerOverflow=on  InputSameDT=on  OutDataTypeStr=Inherit: Same as first input
  Sum11 : Sum  Inputs=-+|  SaturateOnIntegerOverflow=on  InputSameDT=on  OutDataTypeStr=Inherit: Same as first input
  Sum12 : Sum  Inputs=|-+  SaturateOnIntegerOverflow=on  InputSameDT=on  OutDataTypeStr=Inherit: Same as first input
  Sum8 : Sum  Inputs=|++  SaturateOnIntegerOverflow=on  InputSameDT=on  OutDataTypeStr=Inherit: Same as first input
  Sum9 : Sum  Inputs=-+|  SaturateOnIntegerOverflow=on  InputSameDT=on  OutDataTypeStr=Inherit: Same as first input
  Pitch Demand : Outport  InitialOutput=0
  wires:
  Kg/1 -> Sum12/2, "Demand limits "/1
  Gain Scheduled Coefficients Alpha/1("Kg ") -> Kg/1
  Gain Scheduled Coefficients Alpha/3("K ") -> Ka/1
  Gain Scheduled Coefficients Alpha/2("KI ") -> KI/1
  Anti-Windup Gain/1 -> Sum11/1
  Sum8/1 -> Kg/2
  Integrator/1 -> Sum8/1
  Sum11/1 -> Integrator/1
  Product6/1 -> Sum9/1
  Sum9/1 -> Ka/2
  Sum10/1 -> KI/2
  KI/1 -> Sum11/2
  Sum12/1 -> Anti-Windup Gain/1
  "Demand limits "/1 -> Sum12/1, Pitch Demand/1, Scope/1
  Gain Scheduled Coefficients Alpha/4("Ka ") -> Product6/1
  Ka/1 -> Sum10/1
  Gain/1 -> Sum9/2
  Gain1/1 -> Product6/2
  Alpha/1 -> Gain Scheduled Coefficients Alpha/1(Alpha)
  Mach/1 -> Gain Scheduled Coefficients Alpha/2(Mach)
  Ay_m/1 -> Gain1/1
  Ay_d/1 -> Gain/1
  wz_m/1 -> Sum10/2, Sum8/2

== system aeromissile_la/Autopilot/Roll Autopilot ==
  gamma_m : Inport
  wx_m : Inport  Port=2
  "Demand limits " : Saturate  UpperLimit=fin_max  LowerLimit=fin_min
  Integrator1 : Integrator
  KIgamma : Gain  Gain=0.1  SaturateOnIntegerOverflow=on  OutDataTypeStr=Inherit: Same as input  ParamDataTypeStr=Inherit: Same as input
  Kgamma : Gain  Gain=0.1  SaturateOnIntegerOverflow=on  OutDataTypeStr=Inherit: Same as input  ParamDataTypeStr=Inherit: Same as input
  Kwx : Gain  Gain=0.1  SaturateOnIntegerOverflow=on  OutDataTypeStr=Inherit: Same as input  ParamDataTypeStr=Inherit: Same as input
  Scope : Scope
  Sum : Sum  Inputs=|-+  SaturateOnIntegerOverflow=on
  Sum2 : Sum  Inputs=+++  SaturateOnIntegerOverflow=on
  gamma_d : Constant  Value=0
  Roll Demand : Outport
  wires:
  gamma_d/1 -> Sum/1
  Sum2/1 -> "Demand limits "/1
  "Demand limits "/1 -> Roll Demand/1, Scope/1
  gamma_m/1 -> Sum/2, Kgamma/1
  Sum/1 -> KIgamma/1
  KIgamma/1 -> Integrator1/1
  Integrator1/1 -> Sum2/1
  Kgamma/1 -> Sum2/2
  wx_m/1 -> Kwx/1
  Kwx/1 -> Sum2/3

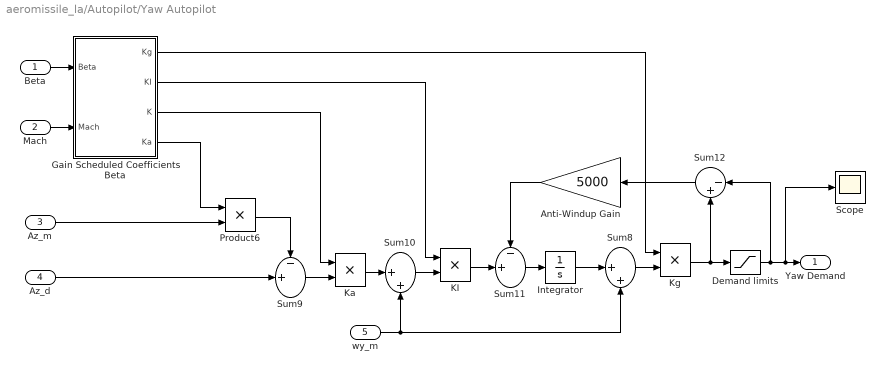
== system aeromissile_la/Autopilot/Yaw Autopilot ==
  Beta : Inport
  Mach : Inport  Port=2
  Az_m : Inport  Port=3
  Az_d : Inport  Port=4
  wy_m : Inport  Port=5
  Anti-Windup Gain : Gain  Gain=5000  SaturateOnIntegerOverflow=on  OutDataTypeStr=Inherit: Same as input  ParamDataTypeStr=Inherit: Same as input
  "Demand limits " : Saturate  UpperLimit=fin_max  LowerLimit=fin_min
  Gain Scheduled Coefficients Beta : Subsystem
  Integrator : Integrator
  KI : Product  SaturateOnIntegerOverflow=on  InputSameDT=on  OutDataTypeStr=Inherit: Same as first input
  Ka : Product  SaturateOnIntegerOverflow=on  InputSameDT=on  OutDataTypeStr=Inherit: Same as first input
  Kg : Product  SaturateOnIntegerOverflow=on  InputSameDT=on  OutDataTypeStr=Inherit: Same as first input
  Product6 : Product  SaturateOnIntegerOverflow=on  InputSameDT=on  OutDataTypeStr=Inherit: Same as first input
  Scope : Scope
  Sum10 : Sum  Inputs=|++  SaturateOnIntegerOverflow=on  InputSameDT=on  OutDataTypeStr=Inherit: Same as first input
  Sum11 : Sum  Inputs=-+|  SaturateOnIntegerOverflow=on  InputSameDT=on  OutDataTypeStr=Inherit: Same as first input
  Sum12 : Sum  Inputs=|-+  SaturateOnIntegerOverflow=on  InputSameDT=on  OutDataTypeStr=Inherit: Same as first input
  Sum8 : Sum  Inputs=|++  SaturateOnIntegerOverflow=on  InputSameDT=on  OutDataTypeStr=Inherit: Same as first input
  Sum9 : Sum  Inputs=-+|  SaturateOnIntegerOverflow=on  InputSameDT=on  OutDataTypeStr=Inherit: Same as first input
  Yaw Demand : Outport  InitialOutput=0
  wires:
  Kg/1 -> Sum12/2, "Demand limits "/1
  Gain Scheduled Coefficients Beta/1("Kg ") -> Kg/1
  Gain Scheduled Coefficients Beta/3("K ") -> Ka/1
  Gain Scheduled Coefficients Beta/2("KI ") -> KI/1
  Anti-Windup Gain/1 -> Sum11/1
  Sum8/1 -> Kg/2
  Integrator/1 -> Sum8/1
  Sum11/1 -> Integrator/1
  Product6/1 -> Sum9/1
  Sum9/1 -> Ka/2
  Sum10/1 -> KI/2
  KI/1 -> Sum11/2
  Sum12/1 -> Anti-Windup Gain/1
  "Demand limits "/1 -> Sum12/1, Yaw Demand/1, Scope/1
  Gain Scheduled Coefficients Beta/4("Ka ") -> Product6/1
  Ka/1 -> Sum10/1
  Beta/1 -> Gain Scheduled Coefficients Beta/1(Beta)
  Mach/1 -> Gain Scheduled Coefficients Beta/2(Mach)
  Az_m/1 -> Product6/2
  Az_d/1 -> Sum9/2
  wy_m/1 -> Sum10/2, Sum8/2

== system aeromissile_la/Start Time/t departure ==
  tS : Inport
  If : If  IfExpression=u1 <= 1.5  ShowElse=off
  If Action Subsystem : Subsystem  TreatAsAtomicUnit=on
  Sum1 : Sum  Inputs=-+  SaturateOnIntegerOverflow=on
  tD : Outport
  wires:
  If/1 -> If Action Subsystem/Action
  If Action Subsystem/1(Out1) -> Sum1/1
  tS/1 -> If Action Subsystem/1(In1), Sum1/2, If/1
  Sum1/1 -> tD/1

== system aeromissile_la/Start Time/t engine ==
  tS : Inport
  If Action Subsystem1 : Subsystem  TreatAsAtomicUnit=on
  If1 : If  IfExpression=u1 <= 3  ShowElse=off
  Sum1 : Sum  Inputs=-+  SaturateOnIntegerOverflow=on
  tE : Outport
  wires:
  If1/1 -> If Action Subsystem1/Action
  If Action Subsystem1/1(Out1) -> Sum1/1
  tS/1 -> If Action Subsystem1/1(In1), Sum1/2, If1/1
  Sum1/1 -> tE/1

== system aeromissile_la/Start Time/t start ==
  S : Inport
  Clock1 : Clock
  If : If  IfExpression=u1 == 0  ShowElse=off
  If Action Subsystem : Subsystem  TreatAsAtomicUnit=on
  Sum2 : Sum  Inputs=-+  SaturateOnIntegerOverflow=on
  tS : Outport
  wires:
  If/1 -> If Action Subsystem/Action
  Clock1/1 -> Sum2/2, If Action Subsystem/1(In1)
  If Action Subsystem/1(Out1) -> Sum2/1
  S/1 -> If/1
  Sum2/1 -> tS/1

== system aeromissile_la/Visualisation/FlightGear Animation ==
  note: Xe
  note: Xg
  Xg : Inport
  Euler : Inport  Port=2
  -h_0 : Constant  Value=-1000
  Demux : Demux  Outputs=2
  Demux1 : Demux  Outputs=3
  Demux2 : Demux  Outputs=3
  Flat Earth to LLA : aerolibtransform2/Flat Earth to LLA  units=Metric (MKS)  ptype=Earth (WGS84)  F=1/298.257223563  R=6378137  LL0=[0 0]  psi=0
  FlightGear Preconfigured 6DoF Animation : aerolibfltsims/FlightGear Preconfigured 6DoF Animation  xFlightGearVersion=v2018.3  DestinationIpAddress=127.0.0.1  DestinationPort=5001  SampleTime=1/60  packetVersion=24
      settings: SourceProductName=Aerospace Blockset
  Mux : Mux  Inputs=6
  Mux1 : Mux  Inputs=3
  Unary Minus1 : UnaryMinus
  wires:
  Unary Minus1/1 -> Mux1/3
  Demux2/2 -> Unary Minus1/1
  Demux2/1 -> Mux1/1
  Xg/1 -> Demux2/1
  Flat Earth to LLA/2 -> Mux/3
  Mux1/1 -> Flat Earth to LLA/1
  Mux/1 -> FlightGear Preconfigured 6DoF Animation/1
  Demux/1 -> Mux/2
  Flat Earth to LLA/1 -> Demux/1
  Demux/2 -> Mux/1
  Demux1/1 -> Mux/4  "phi"
  Demux1/2 -> Mux/5  "theta"
  Demux1/3 -> Mux/6  "psi"
  Demux2/3 -> Mux1/2
  -h_0/1 -> Flat Earth to LLA/2
  Euler/1 -> Demux1/1

== system aeromissile_la/Visualisation/VR Sink Animation ==
  Xg : Inport
  Euler : Inport  Port=2
  Euler to VR Quaternion : Subsystem
  VR Sink : vrlib/VR Sink  InstantiateOnLoad=on  SampleTime=-1  ViewEnable=on  RemoteChange=off  RemoteView=off  FieldsWritten=Cylinder.rotation.4#Cylinder.translation.3  WorldFileName=D:\Matlab6p5Projects\aeromissile\VRMLaeromissile.WRL  WorldDescription=VRMLaeromissile  AutoView=off  VideoDimensions=[]  AllowVariableSize=off
      settings: SourceProductName=Simulink
  wires:
  Euler to VR Quaternion/1(Quaternion) -> VR Sink/1
  Xg/1 -> VR Sink/2
  Euler/1 -> Euler to VR Quaternion/1(Euler Angles)

== system aeromissile_la/Aeromissile Airframe/6DoF Ru (Euler Angles) Mvar/Euler Angles to Direction Cosine Matrix Ru ==
  Euler Roll Pitch Yaw : Inport
  11 : Fcn  Expr=u(6)*u(5)
  12 : Fcn  Expr=u(2)
  13 : Fcn  Expr=-u(3)*u(5)
  21 : Fcn  Expr=u(1)*u(3)-u(4)*u(6)*u(2)
  22 : Fcn  Expr=u(4)*u(5)
  23 : Fcn  Expr=u(1)*u(6)+u(4)*u(3)*u(2)
  31 : Fcn  Expr=u(4)*u(3)+u(1)*u(6)*u(2)
  32 : Fcn  Expr=-u(1)*u(5)
  33 : Fcn  Expr=u(4)*u(6)-u(1)*u(3)*u(2)
  Mux : Mux  Inputs=2
  Mux2 : Mux  Inputs=9
  Reshape 9x1->3x3 : Reshape  OutputDimensionality=Customize  OutputDimensions=[3,3]
  cos(Euler) : Trigonometry  Operator=cos
  sin(Euler) : Trigonometry
  DCM : Outport  InitialOutput=0
  wires:
  33/1 -> Mux2/9
  23/1 -> Mux2/8
  13/1 -> Mux2/7
  32/1 -> Mux2/6
  22/1 -> Mux2/5
  12/1 -> Mux2/4
  31/1 -> Mux2/3
  21/1 -> Mux2/2
  11/1 -> Mux2/1
  Mux2/1 -> Reshape 9x1->3x3/1
  Reshape 9x1->3x3/1 -> DCM/1
  sin(Euler)/1 -> Mux/1
  cos(Euler)/1 -> Mux/2
  Euler Roll Pitch Yaw/1 -> sin(Euler)/1, cos(Euler)/1
  Mux/1 -> 22/1, 11/1, 21/1, 31/1, 12/1, 32/1, 13/1, 23/1, 33/1

== system aeromissile_la/Aeromissile Airframe/6DoF Ru (Euler Angles) Mvar/dgamma//dt dtheta//dt dpsi//dt ==
  wx wy wz : Inport
  gamma theta psi : Inport  Port=2
  Mux1 : Mux  Inputs=[3 3]
  Mux2 : Mux  Inputs=3
  dgamma/dt : Fcn  Expr=u[1]-u[2]*cos(u[4])*tan(u[5])+u[3]*sin(u[4])*tan(u[5])
  dpsi/dt : Fcn  Expr=u[2]*cos(u[4])/cos(u[5])-u[3]*sin(u[4])/cos(u[5])
  dtheta/dt : Fcn  Expr=u[2]*sin(u[4])+u[3]*cos(u[4])
  dgamma/dt dtheta/dt dpsi/dt : Outport  InitialOutput=0
  wires:
  Mux2/1 -> dgamma/dt dtheta/dt dpsi/dt/1
  dgamma/dt/1 -> Mux2/1
  dtheta/dt/1 -> Mux2/2
  dpsi/dt/1 -> Mux2/3
  gamma theta psi/1 -> Mux1/2
  wx wy wz/1 -> Mux1/1
  Mux1/1 -> dtheta/dt/1, dgamma/dt/1, dpsi/dt/1

== system aeromissile_la/Aeromissile Airframe/6DoF Ru (Euler Angles) Mvar/inertia^(-1)x(M-C) ==
  M-C : Inport
  Product : Product  Multiplication=Matrix(*)  SaturateOnIntegerOverflow=on  OutDataTypeStr=Inherit: Same as first input
  inertia(t)^-1 : Subsystem
  dw/dt : Outport
  wires:
  inertia(t)^-1/1(inertia(t)^-1) -> Product/1
  Product/1 -> dw/dt/1
  M-C/1 -> Product/2

== system aeromissile_la/Aeromissile Airframe/6DoF Ru (Euler Angles) Mvar/inertiaxw ==
  w : Inport
  Product : Product  Multiplication=Matrix(*)  SaturateOnIntegerOverflow=on  OutDataTypeStr=Inherit: Same as first input
  inertia(t) : Subsystem
  B : Outport
  wires:
  Product/1 -> B/1
  w/1 -> Product/2
  inertia(t)/1(inertia(t)) -> Product/1

== system aeromissile_la/Aeromissile Airframe/6DoF Ru (Euler Angles) Mvar/m(t)^-1 ==
  Constant : Constant  Value=mass_0
  Constant1 : Constant  Value=massf
  Constant2 : Constant  Value=q
  Constant3 : Constant  Value=-1
  Math Function : Math  Operator=pow  SaturateOnIntegerOverflow=on
  Product : Product  SaturateOnIntegerOverflow=on  OutDataTypeStr=Inherit: Same as first input
  Scope : Scope
  Sum2 : Sum  Inputs=|+-  SaturateOnIntegerOverflow=on
  Sum4 : Sum  Inputs=|+-  SaturateOnIntegerOverflow=on
  Sum5 : Sum  Inputs=|+-  SaturateOnIntegerOverflow=on
  Switch1 : Switch  Criteria=u2 > Threshold  SaturateOnIntegerOverflow=on
  m(t)^-1 : Outport
  wires:
  Constant2/1 -> Product/1
  [tE] -> Product/2
  Constant1/1 -> Sum2/1, Sum4/2
  Product/1 -> Sum2/2, Sum5/2
  Sum2/1 -> Switch1/2
  Sum4/1 -> Switch1/3
  Constant/1 -> Sum5/1, Sum4/1
  Sum5/1 -> Switch1/1
  Switch1/1 -> Scope/1, Math Function/1  "m(t)"
  Constant3/1 -> Math Function/2
  Math Function/1 -> m(t)^-1/1

== system aeromissile_la/Aeromissile Airframe/6DoF Ru (Euler Angles) Mvar/transform to Inertial axes  ==
  x y z : Inport
  transform coefficients : Inport  Port=2
  Product : Product  Multiplication=Matrix(*)  SaturateOnIntegerOverflow=on  InputSameDT=on  OutDataTypeStr=Inherit: Same as first input
  Vg : Outport  InitialOutput=0
  wires:
  Product/1 -> Vg/1
  transform coefficients/1 -> Product/1
  x y z/1 -> Product/2

== system aeromissile_la/Aeromissile Airframe/Aerodynamic Coefficients/Actuator Increments ==
  note: rudder actuators
  note: cx_el
  note: cy_el
  note: cz_el
  note: mx_el
  note: my_el
  note: mz_el
  note: aileron actuators
  Actuator Deflections : Inport
  Demux : Demux  Outputs=3
  Mux : Mux  Inputs=6
  cx : Gain  Gain=0  SaturateOnIntegerOverflow=on  OutDataTypeStr=Inherit: Same as input  ParamDataTypeStr=Inherit: Same as input
  cy : Gain  Gain=cy_el  SaturateOnIntegerOverflow=on  OutDataTypeStr=Inherit: Same as input  ParamDataTypeStr=Inherit: Same as input
  cz : Gain  Gain=cz_el  SaturateOnIntegerOverflow=on  OutDataTypeStr=Inherit: Same as input  ParamDataTypeStr=Inherit: Same as input
  mx : Gain  Gain=mx_el  SaturateOnIntegerOverflow=on  OutDataTypeStr=Inherit: Same as input  ParamDataTypeStr=Inherit: Same as input
  my : Gain  Gain=my_el  SaturateOnIntegerOverflow=on  OutDataTypeStr=Inherit: Same as input  ParamDataTypeStr=Inherit: Same as input
  mz : Gain  Gain=mz_el  SaturateOnIntegerOverflow=on  OutDataTypeStr=Inherit: Same as input  ParamDataTypeStr=Inherit: Same as input
  Actuator Coeffs : Outport  InitialOutput=0
  wires:
  cx/1 -> Mux/1
  my/1 -> Mux/5
  cz/1 -> Mux/3
  cy/1 -> Mux/2
  mx/1 -> Mux/4
  mz/1 -> Mux/6
  Actuator Deflections/1 -> Demux/1
  Demux/1 -> cx/1, cy/1, mz/1  "elevator actuators"
  Demux/2 -> cz/1, my/1
  Mux/1 -> Actuator Coeffs/1
  Demux/3 -> mx/1

== system aeromissile_la/Aeromissile Airframe/Aerodynamic Coefficients/Body Rate Damping ==
  note: mx_wx
  note: my_wy
  note: mz_wz
  wx,wy,wz : Inport
  Demux : Demux  Outputs=3
  Mux : Mux  Inputs=6
  cx : Constant  Value=0
  cy : Constant  Value=0
  cz : Constant  Value=0
  mx : Gain  Gain=mx_wx  SaturateOnIntegerOverflow=on  OutDataTypeStr=Inherit: Same as input  ParamDataTypeStr=Inherit: Same as input
  my : Gain  Gain=my_wy  SaturateOnIntegerOverflow=on  OutDataTypeStr=Inherit: Same as input  ParamDataTypeStr=Inherit: Same as input
  mz : Gain  Gain=mz_wz  SaturateOnIntegerOverflow=on  OutDataTypeStr=Inherit: Same as input  ParamDataTypeStr=Inherit: Same as input
  Damping Coeffs : Outport  InitialOutput=0
  wires:
  my/1 -> Mux/5
  mx/1 -> Mux/4
  mz/1 -> Mux/6
  wx,wy,wz/1 -> Demux/1
  Demux/1 -> mx/1  "wx"
  Demux/2 -> my/1  "wy"
  Demux/3 -> mz/1  "wz"
  cx/1 -> Mux/1
  cy/1 -> Mux/2
  cz/1 -> Mux/3
  Mux/1 -> Damping Coeffs/1
